simulink model "TwoTanks_NL_2018a"  (R2018a)
settings: Solver=FixedStepAuto  StartTime=0.0  StopTime=tfinal  FixedStep=dt  RelTol=1e-3
values from neighbouring files (symbols this model uses):
  a1 = 0.0190125110732    [GWO_workspace.mat]    (also in NGWO_TwoTanks_FO.m; SBAIN_2TANKS.m; TwoTanks_FO_main.m; TwoTanks_NL_main.m)
  a2 = 0.594107643424    [GWO_workspace.mat]    (also in NGWO_TwoTanks_FO.m = num2/den2; SBAIN_2TANKS.m = num2/den2; TwoTanks_FO_main.m = num2/den2; TwoTanks_NL_main.m = num2/den2)
  a3 = 0.0893725569407    [GWO_workspace.mat]    (also in NGWO_TwoTanks_FO.m = num3/den3; SBAIN_2TANKS.m = num3/den3; TwoTanks_FO_main.m = num3/den3; TwoTanks_NL_main.m = num3/den3)
  a4 = 0.0670294177055    [GWO_workspace.mat]    (also in NGWO_TwoTanks_FO.m = num4/den4; SBAIN_2TANKS.m = num4/den4; TwoTanks_FO_main.m = num4/den4; TwoTanks_NL_main.m = num4/den4)
  h10 = 0.25    [GWO_workspace.mat]    (also in NGWO_TwoTanks_FO.m; SBAIN_2TANKS.m; TwoTanks_FO_main.m; TwoTanks_NL_main.m)
  h20 = 0.25    [GWO_workspace.mat]    (also in NGWO_TwoTanks_FO.m; SBAIN_2TANKS.m; TwoTanks_FO_main.m; TwoTanks_NL_main.m)
settings Model: Creator=joniram-XPS  LastModifiedBy=joniram-XPS
settings DataIOCC: ReturnWorkspaceOutputs=on
settings SFSimCC: SimUseLocalCustomCode=on
settings RTWCC: RTWUseLocalCustomCode=on

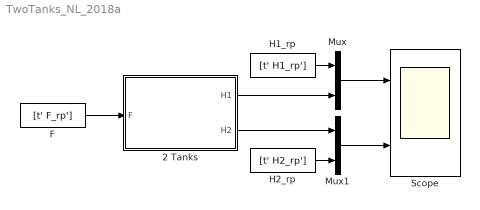
== system TwoTanks_NL_2018a ==
  2 Tanks : Subsystem
  F : FromWorkspace  VariableName=[t' F_rp']  SampleTime=0  OutputAfterFinalValue=Holding final value
  H1_rp : FromWorkspace  VariableName=[t' H1_rp']  SampleTime=0  OutputAfterFinalValue=Holding final value
  H2_rp : FromWorkspace  VariableName=[t' H2_rp']  SampleTime=0  OutputAfterFinalValue=Holding final value
  Mux : Mux  Inputs=2
  Mux1 : Mux  Inputs=2
  Scope : Scope  NumInputPorts=2
  wires:
  F/1 -> 2 Tanks/1(F)
  H1_rp/1 -> Mux/1
  2 Tanks/1(H1) -> Mux/2
  H2_rp/1 -> Mux1/2
  2 Tanks/2(H2) -> Mux1/1
  Mux1/1 -> Scope/2
  Mux/1 -> Scope/1

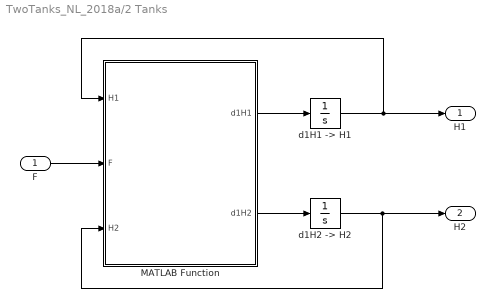
== system TwoTanks_NL_2018a/2 Tanks ==
  F : Inport
  MATLAB Function : MATLAB Function  TreatAsAtomicUnit=on
  "d1H1 -> H1" : Integrator  InitialCondition=h10  LimitOutput=on  LowerSaturationLimit=0
  "d1H2 -> H2" : Integrator  InitialCondition=h20  LimitOutput=on  LowerSaturationLimit=0
  H1 : Outport
  H2 : Outport  Port=2
  wires:
  MATLAB Function/1(d1H1) -> "d1H1 -> H1"/1
  "d1H1 -> H1"/1 -> H1/1, MATLAB Function/1(H1)
  MATLAB Function/2(d1H2) -> "d1H2 -> H2"/1
  F/1 -> MATLAB Function/2(F)
  "d1H2 -> H2"/1 -> H2/1, MATLAB Function/3(H2)

== matlab function TwoTanks_NL_2018a/2 Tanks/MATLAB Function ==
  data: H1 input; F input; d1H1 output; H2 input; d1H2 output; a1 parameter; a2 parameter; a3 parameter; a4 parameter
function [d1H1, d1H2] = TwoTanks(H1, F, H2, a1, a2, a3, a4)
  
  % Sistema Dinâmico 
    d1H1 = a1*F - a2*sqrt(H1);
    
    d1H2 = a3*(sqrt(H1)/(H2^2)) - a4*(1/(H2^1.5));
